simulink model "subtask2_110107589"  (R2023b)
settings: Solver=FixedStepDiscrete  StartTime=0.0  StopTime=(12+392)*8-1  RelTol=1e-3
settings Model: Creator=gowrav -local  LastModifiedBy=AMEY THAKUR

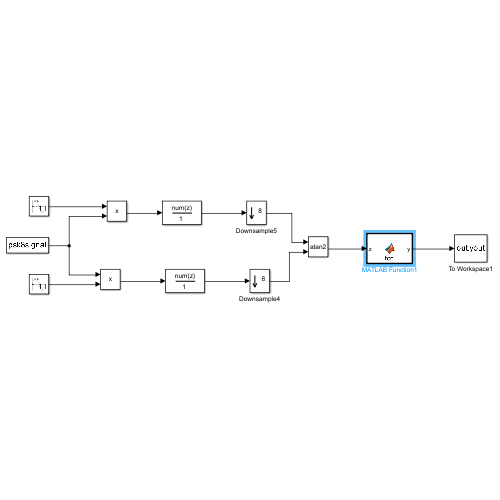
[thumbnail: Simulink's stored preview of the top-level diagram]
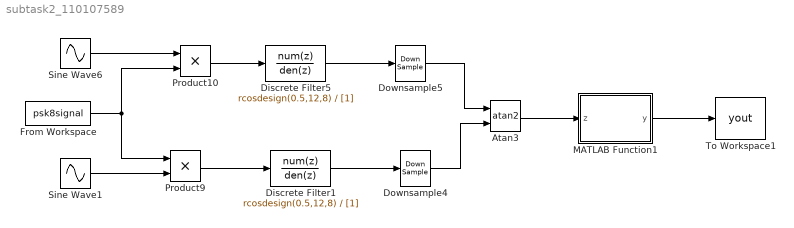
== system subtask2_110107589 ==
  Atan3 : Trigonometry  Operator=atan2
  Discrete Filter1 : DiscreteFilter  Numerator=rcosdesign(0.5,12,8)  Denominator=[1]
  Discrete Filter5 : DiscreteFilter  Numerator=rcosdesign(0.5,12,8)  Denominator=[1]
  Downsample4 : DownSample  N=8  RateOptions=Allow multirate processing
  Downsample5 : DownSample  N=8  RateOptions=Allow multirate processing
  From Workspace : FromWorkspace  VariableName=psk8signal  SampleTime=1
  MATLAB Function1 : MATLAB Function  TreatAsAtomicUnit=on
  Product10 : Product
  Product9 : Product
  Sine Wave1 : Sin  Amplitude=sqrt(2)  Frequency=0.5*pi  Phase=pi/2  SampleTime=1
  Sine Wave6 : Sin  Amplitude=-sqrt(2)  Frequency=0.5*pi  SampleTime=1
  To Workspace1 : ToWorkspace  VariableName=yout  SampleTime=-1
      settings: Save2DSignal=2-D array (concatenate along first dimension)
  wires:
  Sine Wave1/1 -> Product9/2
  Downsample5/1 -> Atan3/1
  Downsample4/1 -> Atan3/2
  Product9/1 -> Discrete Filter1/1
  MATLAB Function1/1(y) -> To Workspace1/1
  Discrete Filter5/1 -> Downsample5/1
  Sine Wave6/1 -> Product10/1
  From Workspace/1 -> Product9/1, Product10/2
  Atan3/1 -> MATLAB Function1/1(z)
  Discrete Filter1/1 -> Downsample4/1
  Product10/1 -> Discrete Filter5/1

== matlab function subtask2_110107589/MATLAB Function1 ==
  data: z input; y output
function y = fcn(z)
y = zeros(size(z));
for i=1:length(z)
    if z(i)>=-(pi/8) && z(i)<(pi/8)
        y(i)=0;
    elseif z(i)>=(-3*(pi/8)) && z(i)<(-(pi/8))
        y(i) = 4;
    elseif z(i)>=(-7*(pi/8)) && z(i)<(-5*(pi/8))
        y(i) = 7;
    elseif z(i)>= 3*pi/8 && z(i)< 5*(pi/8)
        y(i)=3;
    elseif z(i)>= 5*pi/8 && z(i)< 7*(pi/8)
        y(i)=2;
    elseif z(i)>= pi/8 && z(i)< 3*(pi/8)
        y(i)=1;
    elseif z(i)>= -5*pi/8 && z(i)< -3*(pi/8)
        y(i)=5;
    else
        y(i) = 6;
    end
end
